simulink model "Lab5presim"  (R2024b)
settings: Solver=VariableStepAuto  StartTime=0.0  StopTime=200  RelTol=1e-3
values from neighbouring files (symbols this model uses):
  C1 = 10    [Lab5.m]    (also in Lab5pre.m)
  C2 = 0.6    [Lab5.m]    (also in Lab5pre.m)
  K_I = 100    [Lab5pre.m]
  K_P = 100    [Lab5.m]    (also in Lab5pre.m = 200)
settings Model: Creator=camer  LastModifiedBy=camer

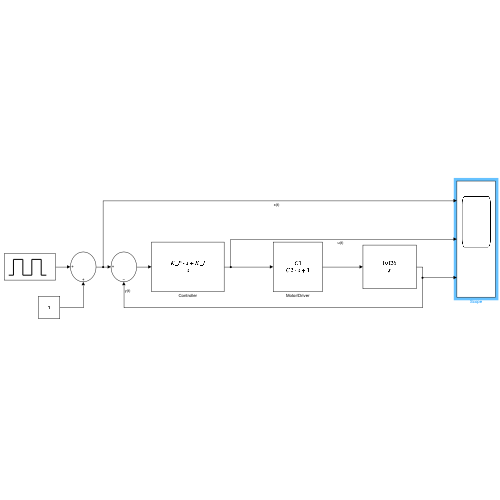
[thumbnail: Simulink's stored preview of the top-level diagram]
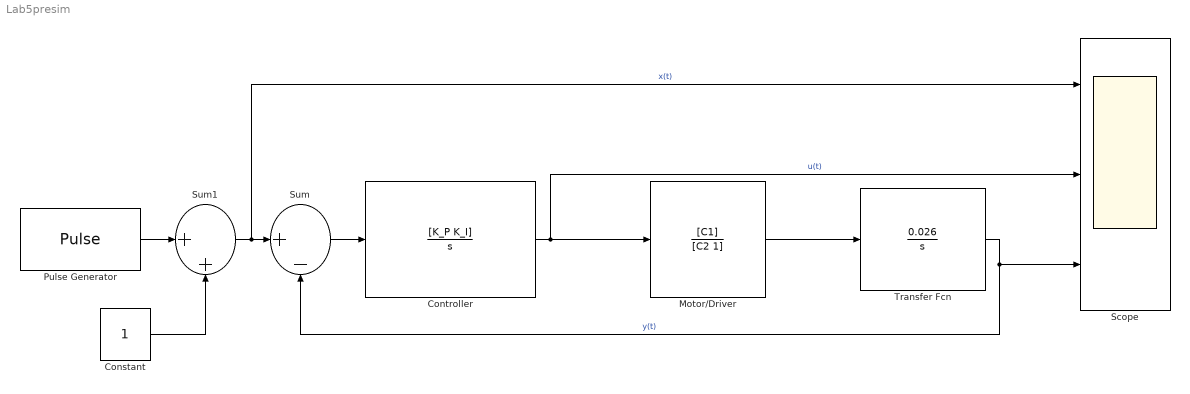
== system Lab5presim ==
  Constant : Constant
  Controller : TransferFcn  Numerator=[K_P K_I]  Denominator=[1 0]
  Motor/Driver : TransferFcn  Numerator=[C1]  Denominator=[C2 1]
  Pulse Generator : DiscretePulseGenerator  PulseType=Time based  Amplitude=3  Period=60  PulseWidth=50
  Scope : Scope  NumInputPorts=3
  Sum : Sum  Inputs=|+-
  Sum1 : Sum  Inputs=|++
  Transfer Fcn : TransferFcn  Numerator=[0.026]  Denominator=[1 0]
  wires:
  Motor/Driver/1 -> Transfer Fcn/1
  Sum/1 -> Controller/1
  Controller/1 -> Motor/Driver/1, Scope/2  "u(t)"
  Transfer Fcn/1 -> Sum/2, Scope/3  "y(t)"
  Sum1/1 -> Scope/1, Sum/1  "x(t)"
  Constant/1 -> Sum1/2
  Pulse Generator/1 -> Sum1/1
